simulink model "suspension_system"  (R2020b)
settings: Solver=VariableStepAuto  StartTime=0.0  StopTime=100.0  RelTol=1e-3
values from neighbouring files (symbols this model uses):
  b = 10    [data.mat]
  k1 = 100    [data.mat]
  k2 = 125    [data.mat]
  m = 0.01    [data.mat]
  M = 1    [data.mat]
settings Model: Creator=JAGRUTI SHINDE  LastModifiedBy=JAGRUTI SHINDE

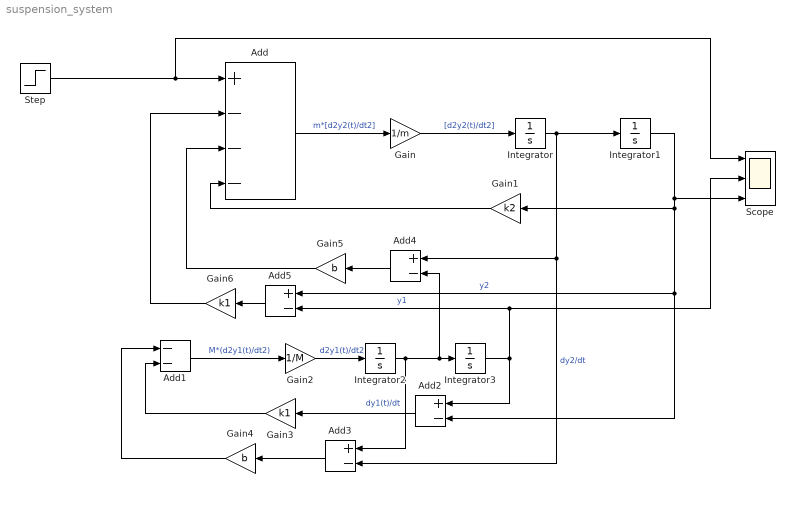
== system suspension_system ==
  Add : Sum  Inputs=+---
  Add1 : Sum  Inputs=--
  Add{2..5} (4 alike) : Sum  Inputs=+-
  Gain : Gain  Gain=1/m
  Gain1 : Gain  Gain=k2
  Gain2 : Gain  Gain=1/M
  Gain3 : Gain  Gain=k1
  Gain4 : Gain  Gain=b
  Gain5 : Gain  Gain=b
  Gain6 : Gain  Gain=k1
  Integrator{,1..3} (4 alike) : Integrator
  Scope : Scope  NumInputPorts=3
  Step : Step  Time=10  SampleTime=0
  wires:
  Step/1 -> Scope/1, Add/1
  Add/1 -> Gain/1  "m*[d2y2(t)/dt2]"
  Gain/1 -> Integrator/1  "[d2y2(t)/dt2]"
  Integrator/1 -> Add4/1, Add3/2, Integrator1/1  "dy2/dt"
  Integrator1/1 -> Scope/3, Add5/1, Add2/2, Gain1/1  "y2"
  Gain1/1 -> Add/4
  Add1/1 -> Gain2/1  "M*(d2y1(t)/dt2)"
  Gain2/1 -> Integrator2/1  "d2y1(t)/dt2"
  Integrator2/1 -> Add3/1, Add4/2, Integrator3/1  "dy1(t)/dt"
  Integrator3/1 -> Scope/2, Add5/2, Add2/1  "y1"
  Add2/1 -> Gain3/1
  Gain3/1 -> Add1/2
  Add3/1 -> Gain4/1
  Gain4/1 -> Add1/1
  Add4/1 -> Gain5/1
  Gain5/1 -> Add/3
  Add5/1 -> Gain6/1
  Gain6/1 -> Add/2
